simulink model "RobotPlant"  (R2023b)
settings: Solver=VariableStepAuto  StartTime=0.0  StopTime=10.0  RelTol=1e-3
values from neighbouring files (symbols this model uses):
  g = 9.81    [RobotParam.m]
  Kd = 0.1    [RobotParam.m]
  L = 1    [RobotParam.m]
  m = 1    [RobotParam.m]
undefined symbols (not defined in the file or in its folder): l
settings Model: Creator=owner  LastModifiedBy=owner

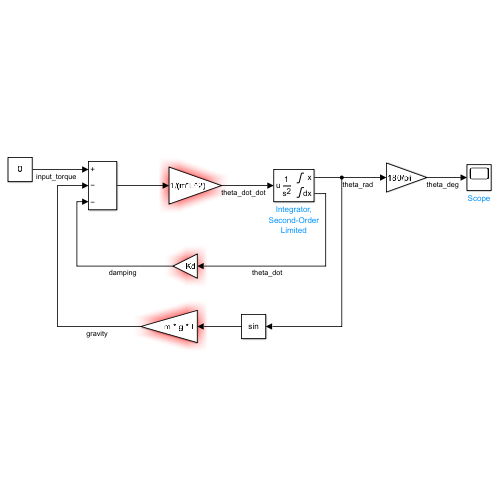
[thumbnail: Simulink's stored preview of the top-level diagram]
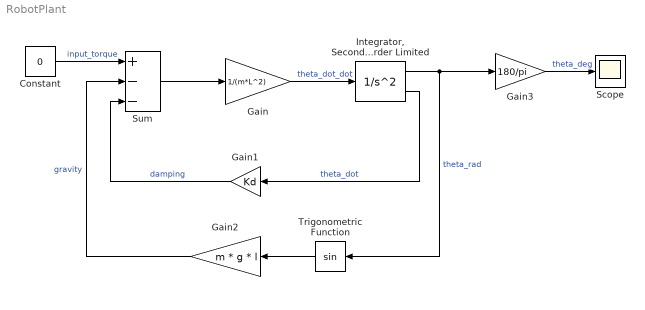
== system RobotPlant ==
  Constant : Constant  Value=0
  Gain : Gain  Gain=1/(m*L^2)
  Gain1 : Gain  Gain=Kd
  Gain2 : Gain  Gain=m * g * l
  Gain3 : Gain  Gain=180/pi
  "Integrator, Second-Order Limited" : SecondOrderIntegrator  LimitX=on  UpperLimitX=1  LowerLimitX=0  LimitDXDT=on
  Scope : Scope
  Sum : Sum  Inputs=+--
  Trigonometric Function : Trigonometry
  wires:
  Constant/1 -> Sum/1  "input_torque"
  Sum/1 -> Gain/1
  Gain/1 -> "Integrator, Second-Order Limited"/1  "theta_dot_dot"
  "Integrator, Second-Order Limited"/1 -> Trigonometric Function/1, Gain3/1  "theta_rad"
  Gain3/1 -> Scope/1  "theta_deg"
  Trigonometric Function/1 -> Gain2/1
  Gain2/1 -> Sum/2  "gravity"
  Gain1/1 -> Sum/3  "damping"
  "Integrator, Second-Order Limited"/2 -> Gain1/1  "theta_dot"
